simulink model "lab6d_dynamics"  (R2013b)
settings: Solver=ode1  StartTime=0.0  StopTime=inf  FixedStep=0.002  RelTol=1e-3
values from neighbouring files (symbols this model uses):
  A = [0 0 0 0 1 -6.81227956989 0 15.4730759462 0 -1.49726820276 0 25.6827715084 ... (16 elements, 4x4)]    [final_ws.mat]    (also in lab6d_runner.m = [0, 1, 0, 0; prelab.m = [0, 1, 0, 0)
  B = [0 1.52258064516 0 -3.45831460894]    [final_ws.mat]    (also in lab6d_runner.m = [0; b_2; 0; b_4]; prelab.m = [0; b_2; 0; b_4])
  C = [1  0  0  0; 0  0  1  0]    [final_ws.mat]    (also in lab6d_runner.m = [1, 0, 0, 0; prelab.m = [1, 0, 1, 0])
  clp = 0.01661    [final_ws.mat]    (also in lab6d_runner.m)
  extract_theta = [0  0  1  0; 0  0  0  1]    [final_ws.mat]    (also in lab6d_runner.m = [0 0 1 0)
  K = [-13.0283303674 -14.7848226904 -48.1649225129 -6.62137714178]    [final_ws.mat]    (also in lab6d_runner.m = [-13.0283303673756 -14.7848226904404 -48.1649225128586 -6.62; prelab.m = [-0.236678439946492, 0.0363618665124172, 0.157443234973144, )
  Kpump = 150    [final_ws.mat]    (also in lab6d_runner.m)
  L = [16.1595  -2.3767; 254.9779  -5.4833; 15.7136  21.0282; 180.7737  378.2196]    [final_ws.mat]    (also in lab6d_runner.m = [16.1595   -2.3767)
  start_time = 0.05    [final_ws.mat]    (also in lab6d_runner.m)
  thresh = 0.261799387799    [final_ws.mat]    (also in lab6d_runner.m)
undefined symbols (not defined in the file or in its folder): HIL
libraries: quarc_library x3
settings Model: SimulationMode=external  ExtModeTrigDuration=1000000  Creator=ee128-abc  LastModifiedBy=ee128-abc
settings SolverCC: PositivePriorityOrder=on
settings DataIOCC: LimitDataPoints=off
settings RTWCC: SystemTargetFile=quarc_win64.tlc  TemplateMakefile=quarc_default_tmf  Description=QUARC Win64 Target  ProcessScript=quarc_win64_make_rtw_hook
settings STFCustomTargetCC: TargetPreCompLibLocation=C:\PROGRA~3\QUARC\lib\2013b\win64\release  GeneratePreprocessorConditionals=Disable all  CombineOutputUpdateFcns=on  GRTInterface=off  SystemTargetFile=quarc_win64.tlc
settings GRTTargetCC: TargetPreCompLibLocation=C:\PROGRA~3\QUARC\lib\2013b\win64\release  ParMdlRefBuildCompliant=off  CompOptLevelCompliant=off  ConcurrentExecutionCompliant=off  MatFileLogging=off  ExtMode=on  ExtModeMexFile=quarc_comm

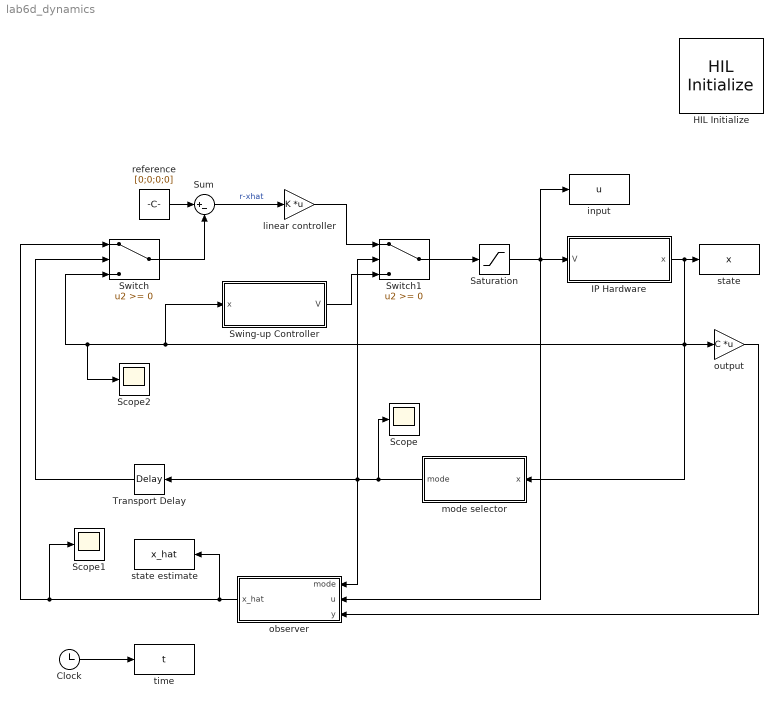
== system lab6d_dynamics ==
  Clock : Clock
  HIL Initialize : quarc_library/Data Acquisition/Generic/Configuration/HIL Initialize  Priority=-99  object_name=HIL-1  board_type=q4  board_number=0  exclusive=off  active=off  hardware_clocks=[0:1]  clock_modes=[0 0]  initial_clock_frequencies=[]  set_clock_params_at_start=on  set_clock_params_at_switch_in=off  set_clock_frequencies_at_start=off  set_clock_frequencies_at_switch_in=off  analog_input_channels=[0:3]  analog_input_maximums=10  analog_input_minimums=-10  set_analog_input_params_at_start=off  set_analog_input_params_at_switch_in=off  analog_output_channels=[0:3]  analog_output_maximums=[10]  analog_output_minimums=[-10]  initial_analog_outputs=[0]  final_analog_outputs=[0]  watchdog_analog_outputs=0  set_analog_output_params_at_start=on  set_analog_output_params_at_switch_in=off  set_analog_outputs_at_start=on  set_analog_outputs_at_switch_in=off  set_analog_outputs_at_terminate=on  set_analog_outputs_at_switch_out=off  set_analog_outputs_on_watchdog=off  digital_input_channels=[]  digital_output_channels=[]  digital_output_configuration=[]  initial_digital_outputs=[1]  final_digital_outputs=[1]  watchdog_digital_outputs=[2]  set_digital_output_params_at_start=off  set_digital_output_params_at_switch_in=off  set_digital_outputs_at_start=on  set_digital_outputs_at_switch_in=off  set_digital_outputs_at_terminate=on  set_digital_outputs_at_switch_out=off  set_digital_outputs_on_watchdog=off  encoder_channels=[0:3]  quadrature=[4]  encoder_filter_frequency=(1/60e-9)/1  initial_encoder_counts=[0]  set_encoder_params_at_start=on  set_encoder_params_at_switch_in=off  set_encoder_counts_at_start=on  set_encoder_counts_at_switch_in=off  pwm_channels=[]  pwm_modes=[0]  pwm_frequency=(1/60e-9)/1024  pwm_configuration=[]  pwm_alignment=[]  pwm_polarity=[]  pwm_leading_deadband=[]  pwm_trailing_deadband=[]  initial_pwm_outputs=[0]  final_pwm_outputs=[0]  watchdog_pwm_outputs=[]  set_pwm_params_at_start=on  set_pwm_params_at_switch_in=off  set_pwm_outputs_at_start=on  set_pwm_outputs_at_switch_in=off  set_pwm_outputs_at_terminate=on  set_pwm_outputs_at_switch_out=off  set_pwm_outputs_on_watchdog=off  other_output_channels=[]  initial_other_outputs=[]  final_other_outputs=[]  watchdog_other_outputs=[]  set_other_outputs_at_start=off  set_other_outputs_at_switch_in=off  set_other_outputs_at_terminate=off  set_other_outputs_at_switch_out=off  set_other_outputs_on_watchdog=off
  "IP Hardware " : Subsystem
  Saturation : Saturate  UpperLimit=6  LowerLimit=-6
  Scope : Scope
      settings: YMin=-1.05  YMax=-0.95
  Scope1 : Scope
      settings: YMin=-12.5  YMax=12.5  SaveName=ScopeData5
  Scope2 : Scope
      settings: YMin=-10  YMax=10  SaveName=ScopeData6
  Sum : Sum  Inputs=|+-
  "Swing-up Controller " : Subsystem
  Switch : Switch
  Switch1 : Switch
  Transport Delay : TransportDelay  DelayTime=.002
  "input " : ToWorkspace  VariableName=u  SampleTime=-1  SaveFormat=Timeseries
  linear controller : Gain  Gain=K  Multiplication=Matrix(K*u)
  "mode selector " : Subsystem
  "observer " : Subsystem
  "output " : Gain  Gain=C  Multiplication=Matrix(K*u)
  "reference " : Constant  Value=[0;0;0;0]
  "state " : ToWorkspace  VariableName=x  SampleTime=-1  SaveFormat=Timeseries
  "state estimate " : ToWorkspace  VariableName=x_hat  SampleTime=-1  SaveFormat=Timeseries
  "time " : ToWorkspace  VariableName=t  SampleTime=-1  SaveFormat=Timeseries
  wires:
  Switch/1 -> Sum/2
  Sum/1 -> linear controller/1  "r-xhat"
  linear controller/1 -> Switch1/1
  Switch1/1 -> Saturation/1
  Saturation/1 -> "observer "/2("u "), "input "/1, "IP Hardware "/1(V)
  "IP Hardware "/1("x ") -> "mode selector "/1("x "), "output "/1, "Swing-up Controller "/1("x "), Scope2/1, Switch/3, "state "/1
  "observer "/1("x_hat ") -> "state estimate "/1, Scope1/1, Switch/1
  "Swing-up Controller "/1("V ") -> Switch1/3
  "mode selector "/1("mode ") -> Scope/1, Transport Delay/1, "observer "/1("mode "), Switch1/2
  Transport Delay/1 -> Switch/2
  "reference "/1 -> Sum/1
  "output "/1 -> "observer "/3("y ")
  Clock/1 -> "time "/1

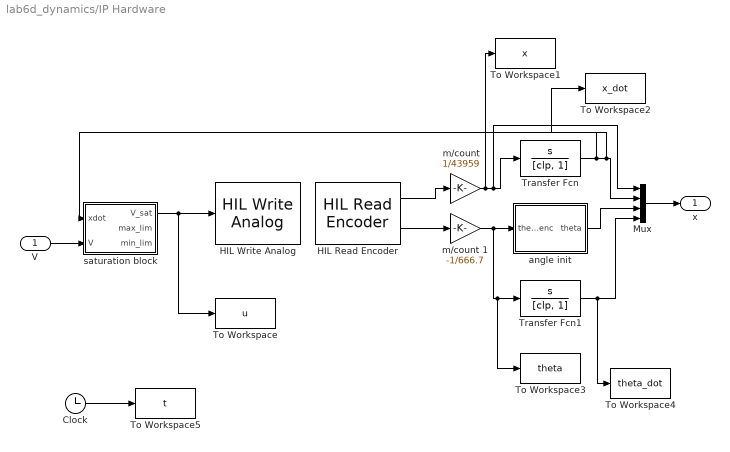
== system lab6d_dynamics/IP Hardware  ==
  V : Inport
  Clock : Clock
  HIL Read Encoder : quarc_library/Data Acquisition/Generic/Immediate I//O/HIL Read Encoder  object_name=HIL-1  channels=[0,1]  sample_time=qc_get_step_size  active=on  vector_output=off  data_type_mode=Inherit via back propagation  data_type=double
  HIL Write Analog : quarc_library/Data Acquisition/Generic/Immediate I//O/HIL Write Analog  object_name=HIL-1  channels=0  sample_time=-1  active=off  vector_input=off
  Mux : Mux
  To Workspace : ToWorkspace  VariableName=u  SampleTime=-1
  To Workspace1 : ToWorkspace  VariableName=x  SampleTime=-1
  To Workspace2 : ToWorkspace  VariableName=x_dot  SampleTime=-1
  To Workspace3 : ToWorkspace  VariableName=theta  SampleTime=-1
  To Workspace4 : ToWorkspace  VariableName=theta_dot  SampleTime=-1
  To Workspace5 : ToWorkspace  VariableName=t  SampleTime=-1
  Transfer Fcn : TransferFcn  Numerator=[1,0]  Denominator=[clp, 1]
  Transfer Fcn1 : TransferFcn  Numerator=[1,0]  Denominator=[clp, 1]
  "angle init " : MATLAB Function  TreatAsAtomicUnit=on
  "m/count " : Gain  Gain=1/43959
  m/count 1 : Gain  Gain=-1/666.7
  "saturation block " : MATLAB Function  TreatAsAtomicUnit=on
  "x " : Outport
  wires:
  V/1 -> "saturation block "/2(V)
  "saturation block "/1(V_sat) -> To Workspace/1, HIL Write Analog/1
  HIL Read Encoder/1 -> "m/count "/1
  HIL Read Encoder/2 -> m/count 1/1
  m/count 1/1 -> To Workspace3/1, Transfer Fcn1/1, "angle init "/1(theta_enc)
  Transfer Fcn1/1 -> To Workspace4/1, Mux/4
  "angle init "/1(theta) -> Mux/3
  "m/count "/1 -> To Workspace1/1, Mux/1, Transfer Fcn/1
  Transfer Fcn/1 -> "saturation block "/1(xdot), To Workspace2/1, Mux/2
  Mux/1 -> "x "/1
  Clock/1 -> To Workspace5/1

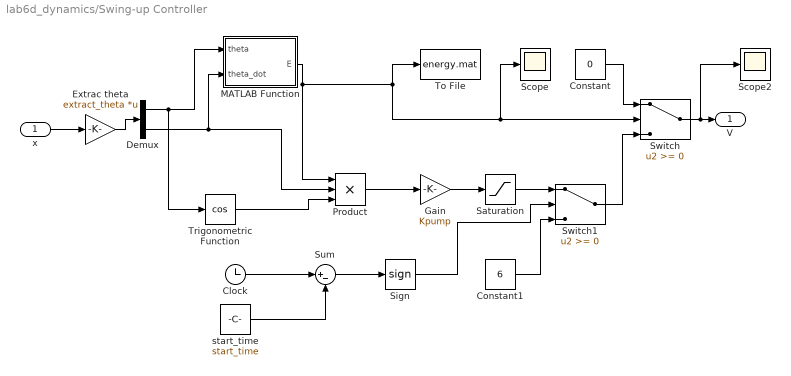
== system lab6d_dynamics/Swing-up Controller  ==
  "x " : Inport
  Clock : Clock
  Constant : Constant  Value=0
  Constant1 : Constant  Value=6
  Demux : Demux  Outputs=2
  Extrac theta : Gain  Gain=extract_theta  Multiplication=Matrix(K*u)
  Gain : Gain  Gain=Kpump
  MATLAB Function : MATLAB Function  TreatAsAtomicUnit=on
  Product : Product  Inputs=3
  Saturation : Saturate  UpperLimit=6  LowerLimit=-6
  Scope : Scope
  Scope2 : Scope
      settings: SaveName=ScopeData2
  Sign : Signum
  Sum : Sum  Inputs=|+-
  Switch : Switch
  Switch1 : Switch
  To File : ToFile  Filename=energy.mat  MatrixName=E
  Trigonometric Function : Trigonometry  Operator=cos
  "start_time " : Constant  Value=start_time
  "V " : Outport
  wires:
  "x "/1 -> Extrac theta/1
  Extrac theta/1 -> Demux/1
  MATLAB Function/1(E) -> Product/1, To File/1, Switch/2, Scope/1
  Constant/1 -> Switch/1
  Switch/1 -> Scope2/1, "V "/1
  Switch1/1 -> Switch/3
  Saturation/1 -> Switch1/1
  Gain/1 -> Saturation/1
  Product/1 -> Gain/1
  Trigonometric Function/1 -> Product/3
  Demux/2 -> MATLAB Function/2(theta_dot), Product/2
  Demux/1 -> Trigonometric Function/1, MATLAB Function/1(theta)
  Constant1/1 -> Switch1/3
  "start_time "/1 -> Sum/2
  Clock/1 -> Sum/1
  Sum/1 -> Sign/1
  Sign/1 -> Switch1/2

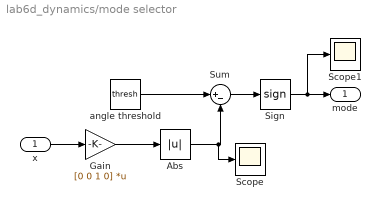
== system lab6d_dynamics/mode selector  ==
  "x " : Inport
  Abs : Abs
  Gain : Gain  Gain=[0 0 1 0]  Multiplication=Matrix(K*u)
  Scope : Scope
      settings: YMin=0.25  YMax=3.25  SaveName=ScopeData3
  Scope1 : Scope
      settings: YMin=1  YMax=1  SaveName=ScopeData4
  Sign : Signum
  Sum : Sum  Inputs=|+-
  "angle threshold " : Constant  Value=thresh
  "mode " : Outport
  wires:
  "x "/1 -> Gain/1
  Gain/1 -> Abs/1
  Abs/1 -> Scope/1, Sum/2
  Sum/1 -> Sign/1
  Sign/1 -> Scope1/1, "mode "/1
  "angle threshold "/1 -> Sum/1

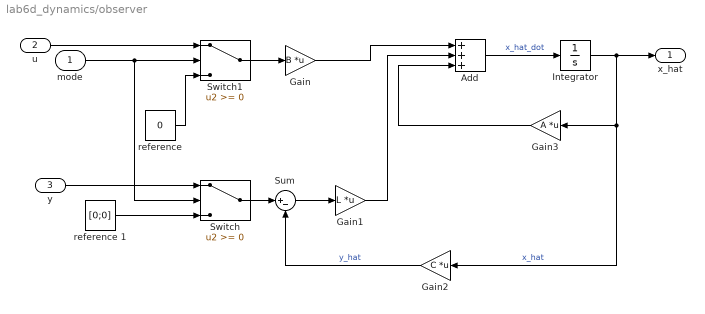
== system lab6d_dynamics/observer  ==
  "mode " : Inport
  "u " : Inport  Port=2
  "y " : Inport  Port=3
  Add : Sum  Inputs=+++
  Gain : Gain  Gain=B  Multiplication=Matrix(K*u)
  Gain1 : Gain  Gain=L  Multiplication=Matrix(K*u)
  Gain2 : Gain  Gain=C  Multiplication=Matrix(K*u)
  Gain3 : Gain  Gain=A  Multiplication=Matrix(K*u)
  Integrator : Integrator
  Sum : Sum  Inputs=|+-
  Switch : Switch
  Switch1 : Switch
  "reference " : Constant  Value=0
  reference 1 : Constant  Value=[0;0]
  "x_hat " : Outport
  wires:
  "u "/1 -> Switch1/1
  "mode "/1 -> Switch/2, Switch1/2
  "reference "/1 -> Switch1/3
  reference 1/1 -> Switch/3
  Switch1/1 -> Gain/1
  Gain2/1 -> Sum/2  "y_hat"
  Sum/1 -> Gain1/1
  Switch/1 -> Sum/1
  Gain/1 -> Add/1
  Gain1/1 -> Add/2
  Add/1 -> Integrator/1  "x_hat_dot"
  Integrator/1 -> Gain2/1, Gain3/1, "x_hat "/1  "x_hat"
  Gain3/1 -> Add/3
  "y "/1 -> Switch/1

== matlab function lab6d_dynamics/IP Hardware /angle init  ==
  data: theta_enc input; theta output
function theta = fcn(theta_enc)
%#codegen
theta = mod(theta_enc, 2*pi) - pi;

== matlab function lab6d_dynamics/IP Hardware /saturation block  ==
  data: xdot input; V_sat output; V input; max_lim output; min_lim output
function [V_sat,max_lim,min_lim] = fcn(xdot, V)
%#codegen
min_lim = -6;
max_lim = 6;

if V < min_lim
    V_sat = min_lim;
elseif V > max_lim
    V_sat = max_lim;
else 
    V_sat = V;
    
end

== matlab function lab6d_dynamics/Swing-up Controller /MATLAB Function ==
  data: theta input; E output; theta_dot input
function E = fcn(theta, theta_dot)
%#codegen
m = .23;
Lp = .3302;
g = 9.81;
J = 4/3*m*Lp^2;


E = 1/2*J*theta_dot^2 + m*g*Lp*(cos(theta)-1);
